simulink subsystem "ProcNav"  (R2020a)
settings: Solver=VariableStepAuto  StartTime=0.0  StopTime=10.0  RelTol=1e-3
undefined symbols (not defined in the file or in its folder): DiscIntNeverNeededParam
libraries: aerolibutil x3, sharedtransform x1
settings Model: Creator=Lamarre  LastModifiedBy=alexemdesgagne

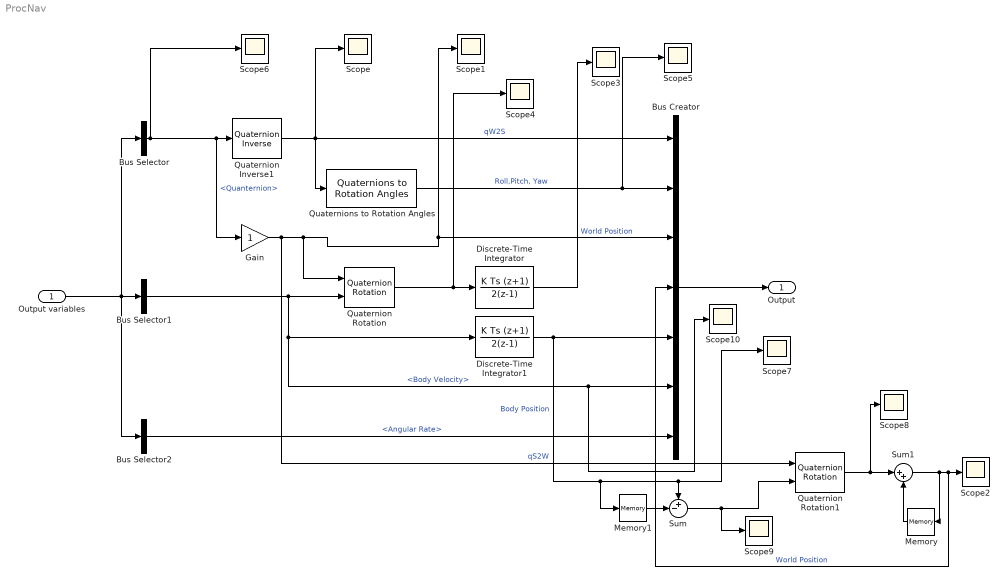
== system ProcNav ==
  Output variables : Inport
  Bus Creator : BusCreator  Inputs=7
  Bus Selector : BusSelector  OutputSignals=Quanternion
  Bus Selector1 : BusSelector  OutputSignals=signal3.Body Velocity
  Bus Selector2 : BusSelector  OutputSignals=Angular Rate
  Discrete-Time Integrator : DiscreteIntegrator  IntegratorMethod=Integration: Trapezoidal  SampleTime=-1  ICPrevOutput=DiscIntNeverNeededParam  ICPrevScaledInput=DiscIntNeverNeededParam
  Discrete-Time Integrator1 : DiscreteIntegrator  IntegratorMethod=Integration: Trapezoidal  SampleTime=-1  ICPrevOutput=DiscIntNeverNeededParam  ICPrevScaledInput=DiscIntNeverNeededParam
  Gain : Gain
  Memory : Memory
  Memory1 : Memory
  Quaternion Inverse1 : aerolibutil/Quaternion Inverse
  Quaternion Rotation : aerolibutil/Quaternion Rotation
  Quaternion Rotation1 : aerolibutil/Quaternion Rotation
  Quaternions to Rotation Angles : sharedtransform/Quaternions to Rotation Angles  rotationOrder=XYZ  aMode=aMode
      settings: SourceProductBaseCode=AE,PW,MT,VE,VP
  Scope{,1..10} (11 alike) : Scope
  Sum : Sum  Inputs=+-|
  Sum1 : Sum  Inputs=|++
  Output : Outport
  wires:
  Quaternions to Rotation Angles/1 -> Scope5/1, Bus Creator/2  "Roll,Pitch, Yaw"
  Bus Selector2/1 -> Bus Creator/7  "<Angular Rate>"
  Output variables/1 -> Bus Selector/1, Bus Selector2/1, Bus Selector1/1
  Bus Selector/1 -> Scope6/1, Quaternion Inverse1/1, Gain/1  "<Quanternion>"
  Discrete-Time Integrator1/1 -> Scope7/1, Sum/1, Memory1/1, Bus Creator/5  "Body Position"
  Quaternion Inverse1/1 -> Bus Creator/1, Scope/1, Quaternions to Rotation Angles/1  "qW2S"
  Discrete-Time Integrator/1 -> Scope3/1  "World Position"
  Bus Creator/1 -> Output/1
  Quaternion Rotation/1 -> Scope4/1, Discrete-Time Integrator/1
  Bus Selector1/1 -> Bus Creator/6, Scope10/1, Discrete-Time Integrator1/1, Quaternion Rotation/2  "<Body Velocity>"
  Gain/1 -> Quaternion Rotation/1, Bus Creator/3, Scope1/1, Quaternion Rotation1/1  "qS2W"
  Memory1/1 -> Sum/2
  Sum/1 -> Quaternion Rotation1/2, Scope9/1
  Quaternion Rotation1/1 -> Sum1/1, Scope8/1
  Sum1/1 -> Scope2/1, Bus Creator/4, Memory/1  "World Position"
  Memory/1 -> Sum1/2
